simulink library "mcs"  (Simulink 8.1)
settings: Solver=ode1  StartTime=0.0  StopTime=Inf  FixedStep=0.001  RelTol=1e-3
PostLoadFcn:
  | , if any(exist('dsrtsu_mdlpostloadfcn', 'file') == [2, 3, 6]), try dsrtsu_mdlpostloadfcn('Execute', bdroot); catch fprintf('Error in PostLoadFcn (dsrtsu_mdlpostloadfcn) for model "%s":\n %s\n', bdroot, lasterr); end, end,
libraries: vpc_new x1, mct x1, sdc x1, tty x1, tdc x1, vip x1
settings Model: DSRTSU_INTERNAL_RTI_VER=450  DSRTSU_INTERNAL_RTI_TYPE=rti1401  RTICANMMDATA=struct('GeneralSetupData',struct('modelroot','D:\ELN150201_TAIWAN\trunk\AdasDragon\software\sw_development\arch\app\ifo','generalsettings',struct('filesettings',struct('destfolder',struct('Name','RTICANMM_FILES','Check',1),'buildfolder',struct('Name','.','Check',1),'AbsDestfolder',struct('Name','D:\ELN150201_TAIWAN\trunk\AdasDragon\software\sw_development\arch\app\ifo\RTICANMM_FILES'),'AbsBuildfolder',struct('Name','D:\ELN150201_TAIWAN\trunk\AdasDragon\software\sw_development\arch\app\ifo'))),'options',struct('addpaths',1,'rmpaths',1,'addtrcexclusion',logical(1),'cannavigator',struct('checkmonitoring',0),'show_usrtrc',0,'use_usrtrc',0),'advanced',struct('options',[1 1 1 1 1 1 1 1 1 1 1 1 1 1 1 1 1 1 1 1 1 1 1 1 1 1 1 1 1 1 1 1 1 1 1 1 1 1 1 1 1 1 1 1 1 1 1 1 1 1 1 1 1 1 1 1 1 1 1 1 1 1 1 1 1 1 1 1 1 1 1 1 1 1 1 1 1 1 1 1 1 1 1 1 1 1 1 1 1 1 1 1 1 1 1 1 1 1 1 1]),'MPSetup',{{}},'modelname','mcs','block','mcs'))  DSRTSU_INTERNAL_RTIFPGA=40  Creator=tescamilla  LastModifiedBy=AT015555

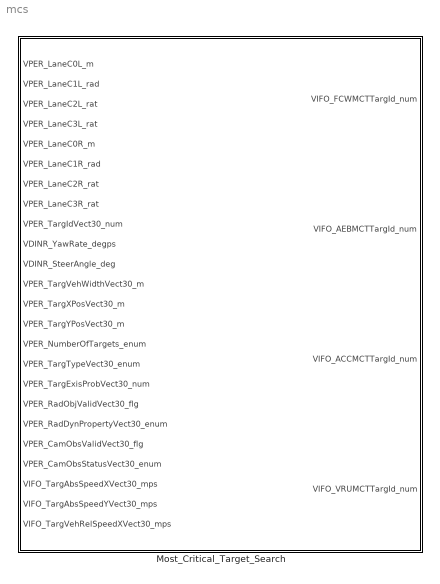
== system mcs ==
  Most_Critical_Target_Search : Subsystem

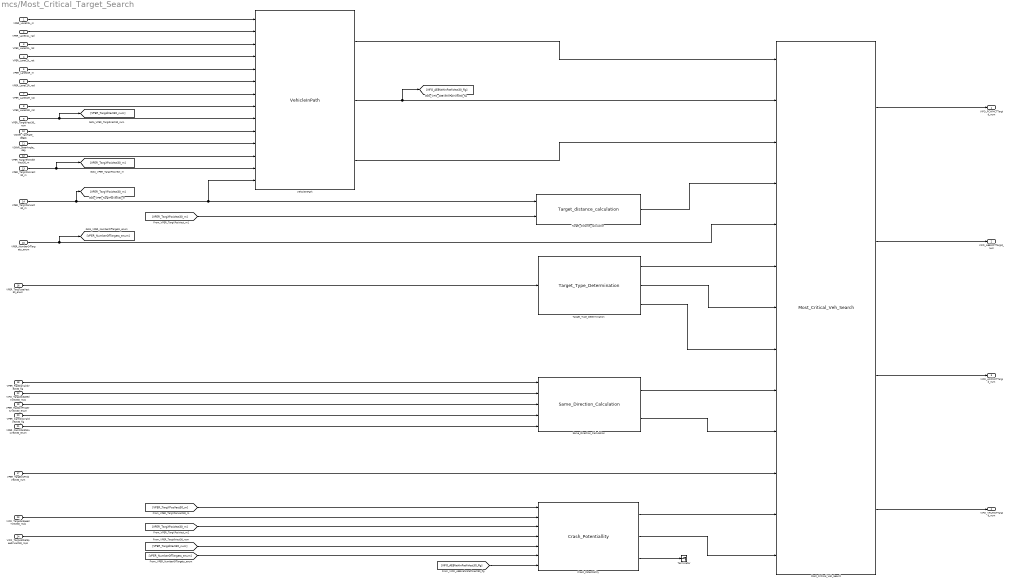
== system mcs/Most_Critical_Target_Search ==
  VPER_LaneC0L_m : Inport
  VPER_LaneC1L_rad : Inport  Port=2
  VPER_LaneC2L_rat : Inport  Port=3
  VPER_LaneC3L_rat : Inport  Port=4
  VPER_LaneC0R_m : Inport  Port=5
  VPER_LaneC1R_rad : Inport  Port=6
  VPER_LaneC2R_rat : Inport  Port=7
  VPER_LaneC3R_rat : Inport  Port=8
  VPER_TargIdVect30_num : Inport  Port=9
  VDINR_YawRate_degps : Inport  Port=10
  VDINR_SteerAngle_deg : Inport  Port=11
  VPER_TargVehWidthVect30_m : Inport  Port=12
  VPER_TargXPosVect30_m : Inport  Port=13
  VPER_TargYPosVect30_m : Inport  Port=14
  VPER_NumberOfTargets_enum : Inport  Port=15
  VPER_TargTypeVect30_enum : Inport  Port=16
  VPER_TargExisProbVect30_num : Inport  Port=17
  VPER_RadObjValidVect30_flg : Inport  Port=18
  VPER_RadDynPropertyVect30_enum : Inport  Port=19
  VPER_CamObsValidVect30_flg : Inport  Port=20
  VPER_CamObsStatusVect30_enum : Inport  Port=21
  VIFO_TargAbsSpeedXVect30_mps : Inport  Port=22
  VIFO_TargAbsSpeedYVect30_mps : Inport  Port=23
  VIFO_TargVehRelSpeedXVect30_mps : Inport  Port=24
  Crash_Potentiallity : vpc_new/Crash_Potentiallity
  Most_Critical_Veh_Search : mct/Most_Critical_Veh_Search
  Same_Direction_Calculation : sdc/Same_Direction_Calculation
  Target_Type_Determination : tty/Target_Type_Determination
  Target_distance_calculation : tdc/Target_distance_calculation
  Terminator : Terminator
  VehicleInPath : vip/VehicleInPath
  VIFO_FCWMCTTargId_num : Outport
  VIFO_AEBMCTTargId_num : Outport  Port=2
  VIFO_ACCMCTTargId_num : Outport  Port=3
  VIFO_VRUMCTTargId_num : Outport  Port=4
  wires:
  Crash_Potentiallity/3 -> Terminator/1
  Crash_Potentiallity/2 -> Most_Critical_Veh_Search/13
  VPER_LaneC3R_rat/1 -> VehicleInPath/8
  VPER_LaneC2R_rat/1 -> VehicleInPath/7
  VPER_LaneC1R_rad/1 -> VehicleInPath/6
  VPER_LaneC0R_m/1 -> VehicleInPath/5
  VPER_LaneC3L_rat/1 -> VehicleInPath/4
  VPER_LaneC2L_rat/1 -> VehicleInPath/3
  VPER_LaneC1L_rad/1 -> VehicleInPath/2
  VPER_LaneC0L_m/1 -> VehicleInPath/1
  [VPER_NumberOfTargets_enum] -> Crash_Potentiallity/6
  [VPER_TargIdVect30_num] -> Crash_Potentiallity/5
  [VIFO_AEBVehInPathVect30_flg] -> Crash_Potentiallity/7
  VIFO_TargVehRelSpeedXVect30_mps/1 -> Crash_Potentiallity/4
  VIFO_TargAbsSpeedYVect30_mps/1 -> Crash_Potentiallity/2
  [VPER_TargYPosVect30_m] -> Crash_Potentiallity/1
  [VPER_TargXPosVect30_m] -> Crash_Potentiallity/3
  Most_Critical_Veh_Search/4 -> VIFO_VRUMCTTargId_num/1
  Crash_Potentiallity/1 -> Most_Critical_Veh_Search/12
  Target_Type_Determination/3 -> Most_Critical_Veh_Search/8
  VPER_RadObjValidVect30_flg/1 -> Same_Direction_Calculation/1
  VPER_CamObsStatusVect30_enum/1 -> Same_Direction_Calculation/5
  VPER_CamObsValidVect30_flg/1 -> Same_Direction_Calculation/4
  VPER_RadDynPropertyVect30_enum/1 -> Same_Direction_Calculation/3
  VPER_TargIdVect30_num/1 -> VehicleInPath/9, [VPER_TargIdVect30_num]
  VPER_TargExisProbVect30_num/1 -> Most_Critical_Veh_Search/11
  VIFO_TargAbsSpeedXVect30_mps/1 -> Same_Direction_Calculation/2
  Most_Critical_Veh_Search/1 -> VIFO_FCWMCTTargId_num/1
  Most_Critical_Veh_Search/2 -> VIFO_AEBMCTTargId_num/1
  VPER_NumberOfTargets_enum/1 -> Most_Critical_Veh_Search/5, [VPER_NumberOfTargets_enum]
  VDINR_SteerAngle_deg/1 -> VehicleInPath/11
  [VPER_TargXPosVect30_m] -> Target_distance_calculation/2
  VDINR_YawRate_degps/1 -> VehicleInPath/10
  VPER_TargTypeVect30_enum/1 -> Target_Type_Determination/1
  Target_distance_calculation/1 -> Most_Critical_Veh_Search/4
  VehicleInPath/2 -> [VIFO_AEBVehInPathVect30_flg], Most_Critical_Veh_Search/2
  VehicleInPath/1 -> Most_Critical_Veh_Search/1
  VPER_TargXPosVect30_m/1 -> [VPER_TargXPosVect30_m], VehicleInPath/13
  VPER_TargVehWidthVect30_m/1 -> VehicleInPath/12
  VPER_TargYPosVect30_m/1 -> Target_distance_calculation/1, VehicleInPath/14, [VPER_TargYPosVect30_m]
  Most_Critical_Veh_Search/3 -> VIFO_ACCMCTTargId_num/1
  VehicleInPath/3 -> Most_Critical_Veh_Search/3
  Target_Type_Determination/2 -> Most_Critical_Veh_Search/7
  Target_Type_Determination/1 -> Most_Critical_Veh_Search/6
  Same_Direction_Calculation/1 -> Most_Critical_Veh_Search/9
  Same_Direction_Calculation/2 -> Most_Critical_Veh_Search/10
